simulink model "preview"  (R2019a)
settings: Solver=VariableStepAuto  StartTime=0.0  StopTime=100  RelTol=1e-3
settings Model: Creator=zgz  LastModifiedBy=zgz
settings DataIOCC: ReturnWorkspaceOutputs=off

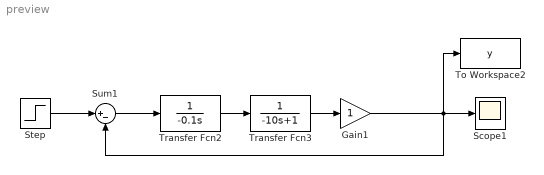
== system preview ==
  Gain1 : Gain
  Scope1 : Scope
  Step : Step  SampleTime=0
  Sum1 : Sum  Inputs=|+-
  To Workspace2 : ToWorkspace  VariableName=y  SampleTime=-1
  Transfer Fcn2 : TransferFcn  Denominator=[-0.1 0]
  Transfer Fcn3 : TransferFcn  Denominator=[-10 1]
  wires:
  Transfer Fcn2/1 -> Transfer Fcn3/1
  Transfer Fcn3/1 -> Gain1/1
  Step/1 -> Sum1/1
  Sum1/1 -> Transfer Fcn2/1
  Gain1/1 -> Scope1/1, To Workspace2/1, Sum1/2
